simulink model "cic_strukturen2"  (Simulink 7.8)
settings: Solver=ode45  StartTime=0.0  StopTime=10.0  RelTol=1e-3
values from neighbouring files (symbols this model uses):
  M = 2    [CFIR_1.m]    (also in block_lms_.m = 16; cic_dezim1.m = ',num2str(M),'; cic_dezim1_.m = ',num2str(M),     '; cic_dezim2.m = ',num2str(M),')
  R = 4    [CFIR_1.m]    (also in cic_dezim1.m = 10; cic_dezim1_.m = ',num2str(R),'; cic_dezim2.m = 10)
libraries: dspsigops x4
settings Model: Creator=svenhoffmann  LastModifiedBy=josef  ExtModeAutoUpdateStatusClock=off
settings OptimizationCC: InlineInvariantSignals=on  InitFltsAndDblsToZero=on
settings DebuggingCC: SaveWithParameterizedLinksMsg=none  SignalResolutionControl=TryResolveAllWithWarning  MultiTaskDSMMsg=warning  MultiTaskCondExecSysMsg=none  StrictBusMsg=None
settings RTWCC: IncludeERTFirstTime=on
settings GRTTargetCC: TargetFcnLib=ansi_tfl_tmw.mat

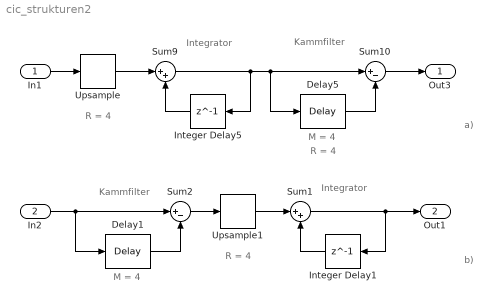
== system cic_strukturen2 ==
  note: b)
  note: R = 4
  note: M = 4
  note: Integrator
  note: Kammfilter
  note: a)
  note: R = 4
  note: R = 4
  note: Integrator
  note: M = 4
  note: Kammfilter
  In1 : Inport
  In2 : Inport  Port=2
  Delay1 : dspsigops/Delay  InputProcessing=Inherited (this choice will be removed - see release notes)  dly_unit=Samples  delay=M  ic_detail=off  dif_ic_for_ch=off  dif_ic_for_dly=off  ic=0  reset_popup=None
  Delay5 : dspsigops/Delay  InputProcessing=Inherited (this choice will be removed - see release notes)  dly_unit=Samples  delay=M*R  ic_detail=off  dif_ic_for_ch=off  dif_ic_for_dly=off  ic=0  reset_popup=None
  Integer Delay1 : Delay  DelayLength=1  InputProcessing=Inherited
  Integer Delay5 : Delay  DelayLength=1  InputProcessing=Inherited
  Sum1 : Sum  Inputs=|++
  Sum10 : Sum  Inputs=|+-
  Sum2 : Sum  Inputs=|+-
  Sum9 : Sum  Inputs=|++
  Upsample : dspsigops/Upsample  N=R  phase=0  InputProcessing=Inherited (this choice will be removed - see release notes)  RateOptions=Allow multirate processing  ic=0  mode=Unused parameter value
  Upsample1 : dspsigops/Upsample  N=R  phase=0  InputProcessing=Inherited (this choice will be removed - see release notes)  RateOptions=Allow multirate processing  ic=0  mode=Unused parameter value
  Out3 : Outport
  Out1 : Outport  Port=2
  wires:
  In2/1 -> Sum2/1, Delay1/1
  In1/1 -> Upsample/1
  Sum9/1 -> Sum10/1, Delay5/1, Integer Delay5/1
  Integer Delay5/1 -> Sum9/2
  Delay5/1 -> Sum10/2
  Sum10/1 -> Out3/1
  Upsample/1 -> Sum9/1
  Upsample1/1 -> Sum1/1
  Sum1/1 -> Integer Delay1/1, Out1/1
  Integer Delay1/1 -> Sum1/2
  Delay1/1 -> Sum2/2
  Sum2/1 -> Upsample1/1
